simulink model "fwv_2020b"  (R2020b)
settings: Solver=ode15s  StartTime=0.0  StopTime=1  RelTol=1e-3  AbsTol=1e-3  EnableMultiTasking=on
model workspace: external: MATLAB File /home/jeff/文档/research/fwvlab/main.m (data not in the file)
values from neighbouring files (symbols this model uses):
  A_D = 1.5    [main.m]    (also in param.m; params.m)
  A_L = 1.8    [main.m]    (also in param.m; params.m)
  c_bar = S/R    (= 0.0357142857143)    [main.m]    (also in param.m = 0.0251327412287; params.m)
  C_D0 = 0.45    [main.m]    (also in param.m; params.m)
  m = 2    [rbf_pid.m]
  r00 = double(int(f,[0,1]))    [main.m]    (also in param.m = 1; params.m = 0.933333333333)
  r11 = double(int(x*f,[0,1]))    [main.m]    (also in param.m = double(int(curv(x)*(x+1/9),0,1)); params.m = 0.481185185185)
  r22 = double(int(x^2*f,[0,1]))    [main.m]    (also in param.m = double(int(curv(x)*(x+1/9)^2,0,1)); params.m = 0.304750617284)
  r33 = double(int(x^3*f,[0,1]))    [main.m]    (also in param.m = double(int(curv(x)*(x+1/9)^3,0,1)); params.m = 0.218568691358)
  r_cp = Rw*r33/r22    [main.m]    (also in param.m; params.m = 0.10758076225)
  rho = 1.205    [main.m]    (also in param.m; params.m)
  Rw = 0.15    [main.m]    (also in param.m = 0.075; params.m)
  z0 = double(int(f^2,[0,1]))    [main.m]
  z1 = double(int(x*f^2,[0,1]))    [main.m]
  z2 = double(int(x^2*f^2,[0,1]))    [main.m]
undefined symbols (not defined in the file or in its folder): X, Y, Z
libraries: sm_lib x45, nesl_utility x38
(part 1 of 2)
settings Model: OrderedModelArguments=off  Creator=jeff  LastModifiedBy=jeff
settings SolverCC: AutoScaleAbsTol=off
settings DataIOCC: LimitDataPoints=on  MaxDataPoints=10000
settings OptimizationCC: LifeSpan=inf
settings DebuggingCC: AllowSymbolicDim=off  SFUnexpectedBacktrackingDiag=warning  SFNoUnconditionalDefaultTransitionDiag=warning  SFExecutionAtInitializationDiag=none  ArithmeticOperatorsInVariantConditions=warning
settings ModelReferenceCC: ModelReferenceMinAlgLoopOccurrences=on
settings SFSimCC: SimUseLocalCustomCode=off  CustomCodeUndefinedFunction=UseInterfaceOnly
settings RTWCC: RTWUseLocalCustomCode=off
settings CodeAppCC: StateflowObjectComments=on
settings GRTTargetCC: TargetLangStandard=C89/C90 (ANSI)
settings ConfigComp: CovMetricSettings=dw  CovSaveCumulativeToWorkspaceVar=on  CovSaveSingleToWorkspaceVar=on  CovExternalEMLEnable=off  CovSFcnEnable=off
settings SimscapeCC: SimscapeLogType=all  SimscapeLogSimulationStatistics=on  SimscapeLogDataHistory=10000

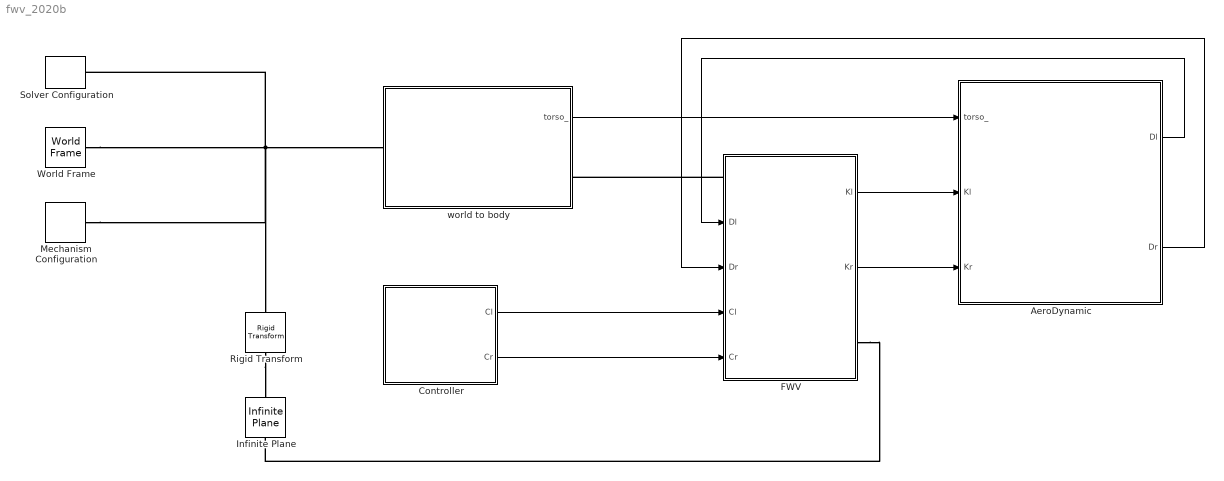
== system fwv_2020b ==
  AeroDynamic : Subsystem
  Controller : Subsystem  mask{f1=20}
  FWV : Subsystem  mask{rho_w=800, stif_rot=5e-3, stif_m=100, damp_m=10}
      settings: PortSchema="{\"entries\":[{\"content\":{\"sides\":[{\"content\":{\"connectorIds\":[\"LConn1\",\"In1\",\"In2\",\"In3\",\"In4\"]},\"type\":\"ConnectorPlacement.EquallySpacedRectSide\",\"uuid\":\"10a6bb1b-48cb-4367-84fe-ad8804c4af6f\"},{\"content\":{\"connectorIds\":[\"Out1\",\"Out2\",\"RConn1\"],\"side\":\"RIGHT\"},\"type\":\"ConnectorPlacement.EquallySpacedRectSide\",\"uuid\":\"a1c0f7ef-a6bf-4be1-8074-dff1a8dbc5c8\"},{\"content\":{\"connectorIds\":[],\"side\":\"TOP\"},\"type\":\"ConnectorPlacement.EquallySpacedRectSide\",\"uuid\":\"74d65e1b-e014-4639-84e4-d97080944fae\"}]},\"type\":\"ConnectorPlacement.EquallySpacedConnector\",\"uuid\":\"e5531aaa-1ccc-4e57-b614-20b26b45530b\"}],\"packageUris\":[\"http://schema.mathworks.com/mf0/Connector/R2020b\"],\"version\":\"1.0\"}"
  Infinite Plane : sm_lib/Curves and Surfaces/Infinite Plane  GraphicType=Rectangle  GraphicPlaneWidth=50  GraphicPlaneWidthUnits=m  GraphicPlaneHeight=50  GraphicPlaneHeightUnits=m  GraphicVisPropType=SimpleVisualProperties  GraphicDiffuseColor=[0.2 0.5 0.8]  GraphicOpacity=1  GraphicSpecularColor=[0.5 0.5 0.5 1.0]  GraphicAmbientColor=[0.15 0.15 0.15 1.0]  GraphicEmissiveColor=[0.0 0.0 0.0 1.0]  GraphicShininess=75
  Mechanism Configuration : sm_lib/Utilities/Mechanism Configuration  UniformGravity=Constant  GravityVector=[0 0 -9.80665]  GravityVectorUnits=m/s^2  GravityUnits=m/s^2  LinearizationDelta=0.001  JointModeTransitionNonlinearIterations=2
  Rigid Transform : sm_lib/Frames and Transforms/Rigid Transform  TranslationMethod=StandardAxis  TranslationStandardOffset=6.5  TranslationLengthUnit=cm  TranslationStandardAxis=-Z  TranslationCartesianOffset=[0 0 0]  TranslationROffset=0  TranslationROffsetUnits=m  TranslationZOffset=0  TranslationZOffsetUnits=m  TranslationThetaOffset=0  TranslationThetaOffsetUnits=deg  RotationMethod=None  RotationAngleUnits=deg  RotationStandardAxis=+Z  RotationAngle=0.0  RotationArbitraryAxis=[0 0 1]  FollAlignAxisA=+X  BaseAlignAxisA=+Y  FollAlignAxisB=+Y  BaseAlignAxisB=+Z  RotationSequenceAxes=FollowerAxes  RotationSequence=XYX  RotationSequenceAngles=[0 0 0]  RotationSequenceAnglesUnits=deg  RotationMatrix=[1 0 0; 0 1 0; 0 0 1]
  Solver Configuration : nesl_utility/Solver Configuration  PhysicalDomain=network_engine_domain  SubClassName=solver  LeftPortType=input  RightPortType=generic  Tones=[]  Harmonics=[]  SimulateNoise=off  Profile=off  UseLocalSampling=off  EnableSwitchedLinearOptims=on  FrequencyDomain=off  UseCCode=off  RelTol=0.001  AbsTol=1e-06  MinStep=1e-09  ToWorkspace=off  RevertToSquareIcSolve=off  NumHomotopyIterations=100  PhasorMode=off  PhasorModeNumHarmonics=1  DoDC=off  ResidualTolerance=1e-09  UseLocalSolver=off  LocalSolverChoice=NE_BACKWARD_EULER_ADVANCER  LocalSolverSampleTime=0.001  DoFixedCost=off  MaxNonlinIter=3  MaxModeIter=2  ComputeImpulses=off  ImpulseIterations=2  LinearAlgebra=Sparse  EquationFormulation=NE_TIME_EF  DelaysMemoryBudget=1024  AutomaticFiltering=on  FilteringTimeConstant=0.001  PartitionStorageMethod=AS_NEEDED  PartitionMemoryBudget=1024  PartitionMethod=FAST
      settings: SourceProductBaseCode=PW,SS
  World Frame : sm_lib/Frames and Transforms/World Frame
  world to body : Subsystem
  wires:
  world to body/1(torso_) -> AeroDynamic/1(torso_)
  FWV/1(Kl) -> AeroDynamic/2(Kl)
  FWV/2(Kr) -> AeroDynamic/3(Kr)
  Controller/1(Cl) -> FWV/3(Cl)
  Controller/2(Cr) -> FWV/4(Cr)
  AeroDynamic/2(Dr) -> FWV/2(Dr)
  AeroDynamic/1(Dl) -> FWV/1(Dl)
  connections:
  Rigid Transform/RConn1 -- Infinite Plane/LConn1
  FWV/RConn1 -- Infinite Plane/RConn1
  FWV/LConn1 -- world to body/RConn1
  World Frame/RConn1 -- world to body/LConn1 -- Mechanism Configuration/RConn1 -- Rigid Transform/LConn1 -- Solver Configuration/RConn1

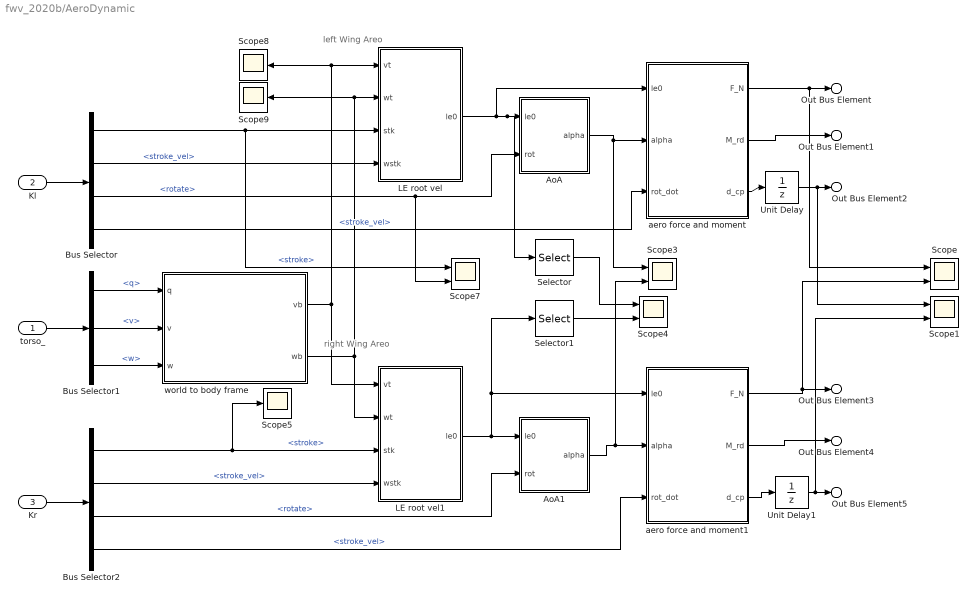
== system fwv_2020b/AeroDynamic ==
  note: right Wing Areo
  note: left Wing Areo
  torso_ : Inport
  Kl : Inport  Port=2
  Kr : Inport  Port=3
  AoA : MATLAB Function  TreatAsAtomicUnit=on
  AoA1 : MATLAB Function  TreatAsAtomicUnit=on
  Bus Selector : BusSelector  OutputSignals=stroke,stroke_vel,rotate,stroke_vel
  Bus Selector1 : BusSelector  OutputSignals=q,v,w
  Bus Selector2 : BusSelector  OutputSignals=stroke,stroke_vel,rotate,stroke_vel
  LE root vel : MATLAB Function  TreatAsAtomicUnit=on
  LE root vel1 : MATLAB Function  TreatAsAtomicUnit=on
  Scope{,1,3..4,7} (5 alike) : Scope  NumInputPorts=2
  Scope5 : Scope
  Scope8 : Scope
  Scope9 : Scope
  Selector : Selector  NumberOfDimensions=2  InputPortWidth=3  IndexOptions=Starting index (dialog),Starting index (dialog)  Indices=2,1  OutputSizes=1,1
  Selector1 : Selector  NumberOfDimensions=2  InputPortWidth=3  IndexOptions=Index vector (dialog),Index vector (dialog)  Indices=2,1  OutputSizes=1,1
  Unit Delay : UnitDelay  InitialCondition=-0.51*c_bar  SampleTime=-1  HasFrameUpgradeWarning=on
  Unit Delay1 : UnitDelay  InitialCondition=-0.51*c_bar  SampleTime=-1  HasFrameUpgradeWarning=on
  aero force and moment : MATLAB Function  TreatAsAtomicUnit=on
  aero force and moment1 : MATLAB Function  TreatAsAtomicUnit=on
  world to body frame : MATLAB Function  TreatAsAtomicUnit=on
  Out Bus Element : Outport  PortName=Dl  Element=FN
  Out Bus Element1 : Outport  PortName=Dl  Element=My
  Out Bus Element2 : Outport  PortName=Dl  Element=d_cp
  Out Bus Element3 : Outport  Port=2  PortName=Dr  Element=FN
  Out Bus Element4 : Outport  Port=2  PortName=Dr  Element=My
  Out Bus Element5 : Outport  Port=2  PortName=Dr  Element=d_cp
  wires:
  AoA/1(alpha) -> Scope3/1, aero force and moment/2(alpha)
  Kl/1 -> Bus Selector/1
  Bus Selector/1 -> Scope7/1, LE root vel/3(stk)  "<stroke>"
  Bus Selector/2 -> LE root vel/4(wstk)  "<stroke_vel>"
  torso_/1 -> Bus Selector1/1
  Bus Selector/3 -> Scope7/2, AoA/2(rot)  "<rotate>"
  Bus Selector1/1 -> world to body frame/1(q)  "<q>"
  Bus Selector1/2 -> world to body frame/2(v)  "<v>"
  Bus Selector1/3 -> world to body frame/3(w)  "<w>"
  world to body frame/1(vb) -> Scope8/1, LE root vel/1(vt), LE root vel1/1(vt)
  world to body frame/2(wb) -> Scope9/1, LE root vel/2(wt), LE root vel1/2(wt)
  LE root vel/1(le0) -> Selector/1, AoA/1(le0), aero force and moment/1(le0)
  aero force and moment/2(M_rd) -> Out Bus Element1/1
  aero force and moment/3(d_cp) -> Unit Delay/1
  Kr/1 -> Bus Selector2/1
  aero force and moment1/2(M_rd) -> Out Bus Element4/1
  aero force and moment1/3(d_cp) -> Unit Delay1/1
  LE root vel1/1(le0) -> Selector1/1, aero force and moment1/1(le0), AoA1/1(le0)
  Bus Selector2/3 -> AoA1/2(rot)  "<rotate>"
  Bus Selector2/1 -> Scope5/1, LE root vel1/3(stk)  "<stroke>"
  Bus Selector2/2 -> LE root vel1/4(wstk)  "<stroke_vel>"
  AoA1/1(alpha) -> Scope3/2, aero force and moment1/2(alpha)
  Bus Selector/4 -> aero force and moment/3(rot_dot)  "<stroke_vel>"
  Bus Selector2/4 -> aero force and moment1/3(rot_dot)  "<stroke_vel>"
  aero force and moment/1(F_N) -> Out Bus Element/1, Scope/1
  aero force and moment1/1(F_N) -> Scope/2, Out Bus Element3/1
  Selector/1 -> Scope4/1
  Selector1/1 -> Scope4/2
  Unit Delay1/1 -> Scope1/2, Out Bus Element5/1
  Unit Delay/1 -> Scope1/1, Out Bus Element2/1

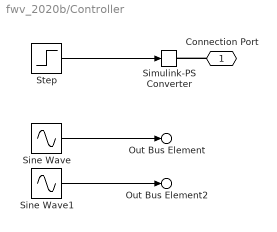
== system fwv_2020b/Controller ==
  Simulink-PS Converter : nesl_utility/Simulink-PS Converter  PhysicalDomain=network_engine_domain  SubClassName=ps_input  LeftPortType=input  RightPortType=output  PseudoPeriodic=off  Frequencies=[]  NoiseDistribution=none  NoiseParameters=[]  Unit=1  AffineConversion=off  FilteringAndDerivatives=provide  SimscapeFilterOrder=1  InputFilterTimeConstant=0.001  UdotUserProvided=0
      settings: SourceProductBaseCode=PW,SS
  Sine Wave : Sin  Amplitude=pi/3  Frequency=f1*2*pi  SampleTime=0
  Sine Wave1 : Sin  Amplitude=pi/3  Frequency=f1*2*pi  SampleTime=0
  Step : Step  Time=0.09  After=-1  SampleTime=0
  Connection Port : PMIOPort  Side=Left
  Out Bus Element : Outport  PortName=Cl  Element=stroke
  Out Bus Element2 : Outport  Port=2  PortName=Cr  Element=stroke
  wires:
  Sine Wave/1 -> Out Bus Element/1
  Sine Wave1/1 -> Out Bus Element2/1
  Step/1 -> Simulink-PS Converter/1
  connections:
  Connection Port/RConn1 -- Simulink-PS Converter/RConn1

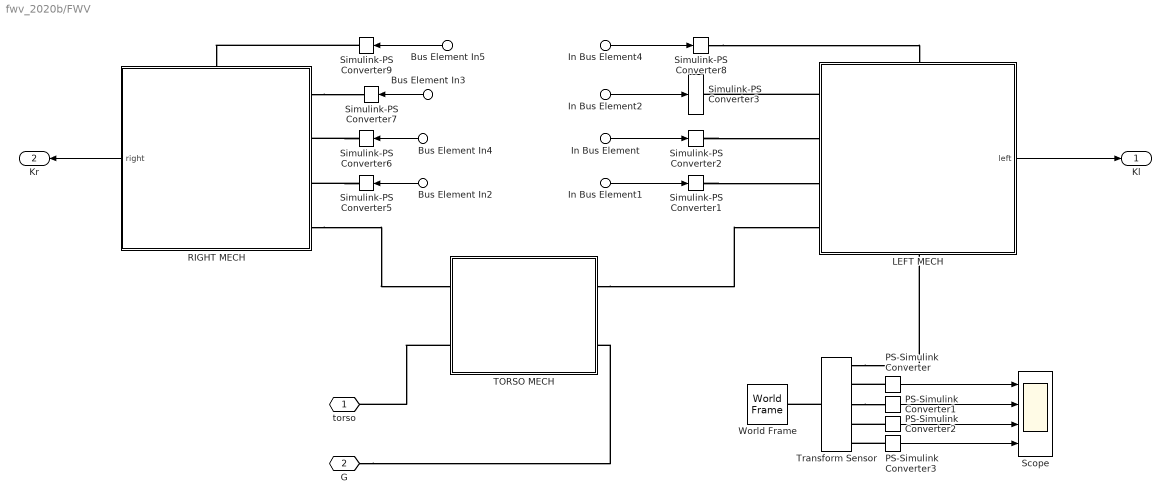
== system fwv_2020b/FWV ==
  In Bus Element : Inport  PortName=Dl  Element=FN
  In Bus Element1 : Inport  PortName=Dl  Element=My
  In Bus Element4 : Inport  PortName=Dl  Element=d_cp
  Bus Element In4 : Inport  Port=2  PortName=Dr  Element=FN
  Bus Element In2 : Inport  Port=2  PortName=Dr  Element=My
  Bus Element In5 : Inport  Port=2  PortName=Dr  Element=d_cp
  In Bus Element2 : Inport  Port=3  PortName=Cl  Element=stroke
  Bus Element In3 : Inport  Port=4  PortName=Cr  Element=stroke
  LEFT MECH : Subsystem
      settings: PortSchema="{\"entries\":[{\"content\":{\"sides\":[{\"content\":{\"connectorIds\":[\"LConn1\",\"LConn2\",\"LConn3\",\"LConn4\"]},\"type\":\"ConnectorPlacement.EquallySpacedRectSide\",\"uuid\":\"3b3bd30c-9c3d-4020-920e-73dfb95645be\"},{\"content\":{\"connectorIds\":[\"Out1\"],\"side\":\"RIGHT\"},\"type\":\"ConnectorPlacement.EquallySpacedRectSide\",\"uuid\":\"6bf80106-81c9-4f1a-b6c7-4ab6b75d5951\"},{\"content\":{\"connectorIds\":[\"LConn5\"],\"side\":\"TOP\"},\"type\":\"ConnectorPlacement.EquallySpacedRectSide\",\"uuid\":\"ce1b4233-3217-452e-b464-d84889ce50ed\"},{\"content\":{\"connectorIds\":[\"RConn1\"],\"side\":\"BOTTOM\"},\"type\":\"ConnectorPlacement.EquallySpacedRectSide\",\"uuid\":\"0b387201-862b-4d94-b297-724f4b58a817\"}]},\"type\":\"ConnectorPlacement.EquallySpacedConnector\",\"uuid\":\"4ad9753c-a95f-426b-a419-920792cb5c12\"}],\"packageUris\":[\"http://schema.mathworks.com/mf0/Connector/R2020b\"],\"version\":\"1.0\"}"
  PS-Simulink Converter{,1..3} (4 alike) : nesl_utility/PS-Simulink Converter  PhysicalDomain=network_engine_domain  SubClassName=ps_output  LeftPortType=input  RightPortType=output  PseudoPeriodic=off  Frequencies=[]  Unit=inherit  AffineConversion=off
      settings: SourceProductBaseCode=PW,SS
  RIGHT MECH : Subsystem
      settings: PortSchema="{\"entries\":[{\"content\":{\"sides\":[{\"content\":{\"connectorIds\":[\"LConn1\",\"LConn2\",\"LConn3\",\"LConn4\"]},\"type\":\"ConnectorPlacement.EquallySpacedRectSide\",\"uuid\":\"3b3bd30c-9c3d-4020-920e-73dfb95645be\"},{\"content\":{\"connectorIds\":[\"Out1\"],\"side\":\"RIGHT\"},\"type\":\"ConnectorPlacement.EquallySpacedRectSide\",\"uuid\":\"6bf80106-81c9-4f1a-b6c7-4ab6b75d5951\"},{\"content\":{\"connectorIds\":[\"LConn5\"],\"side\":\"TOP\"},\"type\":\"ConnectorPlacement.EquallySpacedRectSide\",\"uuid\":\"ce1b4233-3217-452e-b464-d84889ce50ed\"},{\"content\":{\"connectorIds\":[],\"side\":\"BOTTOM\"},\"type\":\"ConnectorPlacement.EquallySpacedRectSide\",\"uuid\":\"e55bd33d-a165-4775-a049-8f5077b03cfa\"}]},\"type\":\"ConnectorPlacement.EquallySpacedConnector\",\"uuid\":\"4ad9753c-a95f-426b-a419-920792cb5c12\"}],\"packageUris\":[\"http://schema.mathworks.com/mf0/Connector/R2020b\"],\"version\":\"1.0\"}"
  Scope : Scope  NumInputPorts=4
  Simulink-PS Converter{1..2,5..9} (7 alike) : nesl_utility/Simulink-PS Converter  PhysicalDomain=network_engine_domain  SubClassName=ps_input  LeftPortType=input  RightPortType=output  PseudoPeriodic=off  Frequencies=[]  NoiseDistribution=none  NoiseParameters=[]  Unit=1  AffineConversion=off  FilteringAndDerivatives=filter  SimscapeFilterOrder=2  InputFilterTimeConstant=0.001  UdotUserProvided=0
      settings: SourceProductBaseCode=PW,SS
  Simulink-PS Converter3 : nesl_utility/Simulink-PS Converter  PhysicalDomain=network_engine_domain  SubClassName=ps_input  LeftPortType=input  RightPortType=output  PseudoPeriodic=off  Frequencies=[]  NoiseDistribution=none  NoiseParameters=[]  Unit=1  AffineConversion=off  FilteringAndDerivatives=filter  SimscapeFilterOrder=2  InputFilterTimeConstant=0.001  UdotUserProvided=2
      settings: SourceProductBaseCode=PW,SS
  TORSO MECH : Subsystem  mask{mu0=0, mu1=0}
  Transform Sensor : sm_lib/Frames and Transforms/Transform Sensor  MeasurementFrame=NonRotatingFollower  SenseAngle=off  SenseAxis=off  SenseAngle1=off  SenseAngle2=off  SenseAngle3=off  SenseQ=off  SenseR=off  SenseOmegaX=on  SenseOmegaY=off  SenseOmegaZ=on  SenseOmega1=off  SenseOmega2=off  SenseOmega3=off  SenseQDot=off  SenseRDot=off  SenseAlphaX=off  SenseAlphaY=off  SenseAlphaZ=off  SenseAlpha1=off  SenseAlpha2=off  SenseAlpha3=off  SenseQDDot=off  SenseRDDot=off  SenseX=off  SenseY=off  SenseZ=off  SenseRad=off  SenseAzim=off  SenseDist=off  SenseInc=off  SenseXDot=on  SenseYDot=off  SenseZDot=on  SenseRadDot=off  SenseAzimDot=off  SenseDistDot=off  SenseIncDot=off  SenseXDDot=off  SenseYDDot=off  SenseZDDot=off  SenseRadDDot=off  SenseAzimDDot=off  SenseDistDDot=off  SenseIncDDot=off
  World Frame : sm_lib/Frames and Transforms/World Frame
  torso : PMIOPort  Side=Left
  G : PMIOPort  Port=2  Side=Right
  Kl : Outport
  Kr : Outport  Port=2
  wires:
  LEFT MECH/1(left) -> Kl/1
  RIGHT MECH/1(right) -> Kr/1
  In Bus Element1/1 -> Simulink-PS Converter1/1
  In Bus Element/1 -> Simulink-PS Converter2/1
  In Bus Element2/1 -> Simulink-PS Converter3/1
  Bus Element In3/1 -> Simulink-PS Converter7/1
  Bus Element In4/1 -> Simulink-PS Converter6/1
  Bus Element In2/1 -> Simulink-PS Converter5/1
  In Bus Element4/1 -> Simulink-PS Converter8/1
  Bus Element In5/1 -> Simulink-PS Converter9/1
  PS-Simulink Converter/1 -> Scope/1
  PS-Simulink Converter1/1 -> Scope/2
  PS-Simulink Converter2/1 -> Scope/3
  PS-Simulink Converter3/1 -> Scope/4
  connections:
  G/RConn1 -- TORSO MECH/RConn2
  TORSO MECH/LConn2 -- torso/RConn1
  TORSO MECH/RConn1 -- LEFT MECH/LConn4
  RIGHT MECH/LConn4 -- TORSO MECH/LConn1
  LEFT MECH/LConn1 -- Simulink-PS Converter3/RConn1
  RIGHT MECH/LConn1 -- Simulink-PS Converter7/RConn1
  Simulink-PS Converter2/RConn1 -- LEFT MECH/LConn2
  Simulink-PS Converter1/RConn1 -- LEFT MECH/LConn3
  Simulink-PS Converter6/RConn1 -- RIGHT MECH/LConn2
  Simulink-PS Converter5/RConn1 -- RIGHT MECH/LConn3
  Simulink-PS Converter8/RConn1 -- LEFT MECH/LConn5
  Simulink-PS Converter9/RConn1 -- RIGHT MECH/LConn5
  Transform Sensor/LConn1 -- World Frame/RConn1
  Transform Sensor/RConn1 -- LEFT MECH/RConn1
  PS-Simulink Converter/LConn1 -- Transform Sensor/RConn2
  Transform Sensor/RConn3 -- PS-Simulink Converter1/LConn1
  PS-Simulink Converter2/LConn1 -- Transform Sensor/RConn4
  PS-Simulink Converter3/LConn1 -- Transform Sensor/RConn5

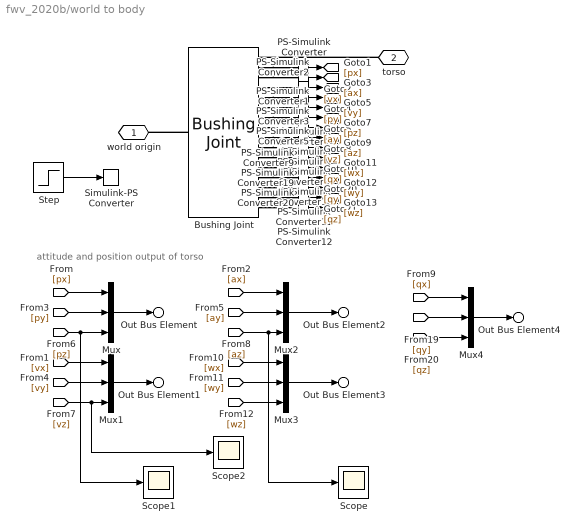
== system fwv_2020b/world to body ==
  note: attitude and position output of torso
  Bushing Joint : sm_lib/Joints/Bushing Joint  JointMode=Normal  SenseConstraintForce=off  SenseConstraintForceX=off  SenseConstraintForceY=off  SenseConstraintForceZ=off  SenseConstraintTorque=off  SenseConstraintTorqueX=off  SenseConstraintTorqueY=off  SenseConstraintTorqueZ=off  SenseTotalForce=off  SenseTotalForceX=off  SenseTotalForceY=off  SenseTotalForceZ=off  SenseTotalTorque=off  SenseTotalTorqueX=off  SenseTotalTorqueY=off  SenseTotalTorqueZ=off  CompositeWrenchDir=FollowerOnBase  CompositeWrenchFrame=BaseFrame  PxEquilibriumPosition=0  PxEquilibriumPositionUnits=m  PxSpringStiffness=0  PxSpringStiffnessUnits=N/m  PxDampingCoefficient=0  PxDampingCoefficientUnits=N/(m/s)  PxTorqueActuationMode=NoTorque  PxMotionActuationMode=ComputedMotion  PxSensePosition=on  PxSenseVelocity=on  PxSenseAcceleration=on  PxSenseTorqueForce=off  PxSenseLowerLimitTorqueForce=off  PxSenseUpperLimitTorqueForce=off  PxLowerLimitSpecify=off  PxLowerLimitBound=-1  PxLowerLimitBoundUnits=m  PxLowerLimitStiffness=1e6  PxLowerLimitStiffnessUnits=N/m  PxLowerLimitDamping=1e3  PxLowerLimitDampingUnits=N/(m/s)  PxLowerLimitTransitionRegionWidth=1e-4  PxLowerLimitTransitionRegionWidthUnits=m  PxUpperLimitSpecify=off  PxUpperLimitBound=1  PxUpperLimitBoundUnits=m  PxUpperLimitStiffness=1e6  PxUpperLimitStiffnessUnits=N/m  PxUpperLimitDamping=1e3  PxUpperLimitDampingUnits=N/(m/s)  PxUpperLimitTransitionRegionWidth=1e-4  PxUpperLimitTransitionRegionWidthUnits=m  PxPositionTargetSpecify=off  PxPositionTargetPriority=High  PxPositionTargetValue=0  PxPositionTargetValueUnits=m  PxVelocityTargetSpecify=off  PxVelocityTargetPriority=High  PxVelocityTargetValue=0  PxVelocityTargetValueUnits=m/s  PyEquilibriumPosition=0  PyEquilibriumPositionUnits=m  PySpringStiffness=0  PySpringStiffnessUnits=N/m  PyDampingCoefficient=0  PyDampingCoefficientUnits=N/(m/s)  PyTorqueActuationMode=NoTorque  PyMotionActuationMode=ComputedMotion  PySensePosition=on  PySenseVelocity=on  PySenseAcceleration=on  PySenseTorqueForce=off  PySenseLowerLimitTorqueForce=off  PySenseUpperLimitTorqueForce=off  PyLowerLimitSpecify=off  PyLowerLimitBound=-1  PyLowerLimitBoundUnits=m  PyLowerLimitStiffness=1e6  PyLowerLimitStiffnessUnits=N/m  PyLowerLimitDamping=1e3  PyLowerLimitDampingUnits=N/(m/s)  PyLowerLimitTransitionRegionWidth=1e-4  PyLowerLimitTransitionRegionWidthUnits=m  PyUpperLimitSpecify=off  PyUpperLimitBound=1  PyUpperLimitBoundUnits=m  PyUpperLimitStiffness=1e6  PyUpperLimitStiffnessUnits=N/m  PyUpperLimitDamping=1e3  PyUpperLimitDampingUnits=N/(m/s)  PyUpperLimitTransitionRegionWidth=1e-4  PyUpperLimitTransitionRegionWidthUnits=m  PyPositionTargetSpecify=off  PyPositionTargetPriority=High  PyPositionTargetValue=0  PyPositionTargetValueUnits=m  PyVelocityTargetSpecify=off  PyVelocityTargetPriority=High  PyVelocityTargetValue=0  PyVelocityTargetValueUnits=m/s  PzEquilibriumPosition=0  PzEquilibriumPositionUnits=m  PzSpringStiffness=0  PzSpringStiffnessUnits=N/m  PzDampingCoefficient=0  PzDampingCoefficientUnits=N/(m/s)  PzTorqueActuationMode=NoTorque  PzMotionActuationMode=ComputedMotion  PzSensePosition=on  PzSenseVelocity=on  PzSenseAcceleration=on  PzSenseTorqueForce=off  PzSenseLowerLimitTorqueForce=off  PzSenseUpperLimitTorqueForce=off  PzLowerLimitSpecify=off  PzLowerLimitBound=-1  PzLowerLimitBoundUnits=m  PzLowerLimitStiffness=1e6  PzLowerLimitStiffnessUnits=N/m  PzLowerLimitDamping=1e3  PzLowerLimitDampingUnits=N/(m/s)  PzLowerLimitTransitionRegionWidth=1e-4  PzLowerLimitTransitionRegionWidthUnits=m  PzUpperLimitSpecify=off  PzUpperLimitBound=1  PzUpperLimitBoundUnits=m  PzUpperLimitStiffness=1e6  PzUpperLimitStiffnessUnits=N/m  PzUpperLimitDamping=1e3  PzUpperLimitDampingUnits=N/(m/s)  PzUpperLimitTransitionRegionWidth=1e-4  PzUpperLimitTransitionRegionWidthUnits=m  PzPositionTargetSpecify=off  PzPositionTargetPriority=High  PzPositionTargetValue=0  PzPositionTargetValueUnits=m  PzVelocityTargetSpecify=off  PzVelocityTargetPriority=High  PzVelocityTargetValue=0  PzVelocityTargetValueUnits=m/s  RxEquilibriumPosition=0  RxEquilibriumPositionUnits=deg  RxSpringStiffness=0  RxSpringStiffnessUnits=N*m/deg  RxDampingCoefficient=0  RxDampingCoefficientUnits=N*m/(deg/s)  RxTorqueActuationMode=NoTorque  RxMotionActuationMode=ComputedMotion  RxSensePosition=on  RxSenseVelocity=on  RxSenseAcceleration=off  RxSenseTorqueForce=off  RxSenseLowerLimitTorqueForce=off  RxSenseUpperLimitTorqueForce=off  RxLowerLimitSpecify=off  RxLowerLimitBound=-90  RxLowerLimitBoundUnits=deg  RxLowerLimitStiffness=1e4  RxLowerLimitStiffnessUnits=N*m/deg  RxLowerLimitDamping=10  RxLowerLimitDampingUnits=N*m/(deg/s)  RxLowerLimitTransitionRegionWidth=0.1  RxLowerLimitTransitionRegionWidthUnits=deg  RxUpperLimitSpecify=off  RxUpperLimitBound=90  RxUpperLimitBoundUnits=deg  RxUpperLimitStiffness=1e4  RxUpperLimitStiffnessUnits=N*m/deg  RxUpperLimitDamping=10  RxUpperLimitDampingUnits=N*m/(deg/s)  RxUpperLimitTransitionRegionWidth=0.1  RxUpperLimitTransitionRegionWidthUnits=deg  RxPositionTargetSpecify=off  RxPositionTargetPriority=High  RxPositionTargetValue=0  RxPositionTargetValueUnits=deg  RxVelocityTargetSpecify=off  RxVelocityTargetPriority=High  RxVelocityTargetValue=0  RxVelocityTargetValueUnits=deg/s  RyEquilibriumPosition=0  RyEquilibriumPositionUnits=deg  RySpringStiffness=0  RySpringStiffnessUnits=N*m/deg  RyDampingCoefficient=0  RyDampingCoefficientUnits=N*m/(deg/s)  RyTorqueActuationMode=NoTorque  RyMotionActuationMode=ComputedMotion  RySensePosition=on  RySenseVelocity=on  RySenseAcceleration=off  RySenseTorqueForce=off  RySenseLowerLimitTorqueForce=off  RySenseUpperLimitTorqueForce=off  RyLowerLimitSpecify=off  RyLowerLimitBound=-90  RyLowerLimitBoundUnits=deg  RyLowerLimitStiffness=1e4  RyLowerLimitStiffnessUnits=N*m/deg  RyLowerLimitDamping=10  RyLowerLimitDampingUnits=N*m/(deg/s)  RyLowerLimitTransitionRegionWidth=0.1  RyLowerLimitTransitionRegionWidthUnits=deg  RyUpperLimitSpecify=off  RyUpperLimitBound=90  RyUpperLimitBoundUnits=deg  RyUpperLimitStiffness=1e4  RyUpperLimitStiffnessUnits=N*m/deg  RyUpperLimitDamping=10  RyUpperLimitDampingUnits=N*m/(deg/s)  RyUpperLimitTransitionRegionWidth=0.1  RyUpperLimitTransitionRegionWidthUnits=deg  RyPositionTargetSpecify=off  RyPositionTargetPriority=High  RyPositionTargetValue=0  RyPositionTargetValueUnits=deg  RyVelocityTargetSpecify=off  RyVelocityTargetPriority=High  RyVelocityTargetValue=0  RyVelocityTargetValueUnits=deg/s  RzEquilibriumPosition=0  RzEquilibriumPositionUnits=deg  RzSpringStiffness=0  RzSpringStiffnessUnits=N*m/deg  RzDampingCoefficient=0  RzDampingCoefficientUnits=N*m/(deg/s)  RzTorqueActuationMode=NoTorque  RzMotionActuationMode=ComputedMotion  RzSensePosition=on  RzSenseVelocity=on  RzSenseAcceleration=off  RzSenseTorqueForce=off  RzSenseLowerLimitTorqueForce=off  RzSenseUpperLimitTorqueForce=off  RzLowerLimitSpecify=off  RzLowerLimitBound=-90  RzLowerLimitBoundUnits=deg  RzLowerLimitStiffness=1e4  RzLowerLimitStiffnessUnits=N*m/deg  RzLowerLimitDamping=10  RzLowerLimitDampingUnits=N*m/(deg/s)  RzLowerLimitTransitionRegionWidth=0.1  RzLowerLimitTransitionRegionWidthUnits=deg  RzUpperLimitSpecify=off  RzUpperLimitBound=90  RzUpperLimitBoundUnits=deg  RzUpperLimitStiffness=1e4  RzUpperLimitStiffnessUnits=N*m/deg  RzUpperLimitDamping=10  RzUpperLimitDampingUnits=N*m/(deg/s)  RzUpperLimitTransitionRegionWidth=0.1  RzUpperLimitTransitionRegionWidthUnits=deg  RzPositionTargetSpecify=off  RzPositionTargetPriority=High  RzPositionTargetValue=45  RzPositionTargetValueUnits=deg  RzVelocityTargetSpecify=off  RzVelocityTargetPriority=High  RzVelocityTargetValue=0  RzVelocityTargetValueUnits=deg/s
  Mux{,1..4} (5 alike) : Mux  Inputs=3
  PS-Simulink Converter{,1..12,19..20} (15 alike) : nesl_utility/PS-Simulink Converter  PhysicalDomain=network_engine_domain  SubClassName=ps_output  LeftPortType=input  RightPortType=output  PseudoPeriodic=off  Frequencies=[]  Unit=inherit  AffineConversion=off
      settings: SourceProductBaseCode=PW,SS
  Scope : Scope
  Scope1 : Scope
  Scope2 : Scope
  Simulink-PS Converter : nesl_utility/Simulink-PS Converter  PhysicalDomain=network_engine_domain  SubClassName=ps_input  LeftPortType=input  RightPortType=output  PseudoPeriodic=off  Frequencies=[]  NoiseDistribution=none  NoiseParameters=[]  Unit=1  AffineConversion=off  FilteringAndDerivatives=provide  SimscapeFilterOrder=1  InputFilterTimeConstant=0.001  UdotUserProvided=0
      settings: SourceProductBaseCode=PW,SS
  Step : Step  Time=0.5  After=0  SampleTime=0
  world origin : PMIOPort  Side=Left
  torso : PMIOPort  Port=2  Side=Right
  Out Bus Element : Outport  PortName=torso_  Element=p
  Out Bus Element1 : Outport  PortName=torso_  Element=v
  Out Bus Element2 : Outport  PortName=torso_  Element=a
  Out Bus Element3 : Outport  PortName=torso_  Element=w
  Out Bus Element4 : Outport  PortName=torso_  Element=q
  wires:
  PS-Simulink Converter10/1 -> [wx]
  PS-Simulink Converter9/1 -> [qx]
  [wz] -> Mux3/3
  [vy] -> Mux1/2
  [px] -> Mux/1
  [ax] -> Mux2/1
  [wx] -> Mux3/1
  PS-Simulink Converter8/1 -> [az]
  [vz] -> Scope2/1, Mux1/3
  Mux1/1 -> Out Bus Element1/1
  [az] -> Scope/1, Mux2/3
  PS-Simulink Converter5/1 -> [ay]
  [vx] -> Mux1/1
  [ay] -> Mux2/2
  PS-Simulink Converter7/1 -> [vz]
  [qy] -> Mux4/2
  [pz] -> Scope1/1, Mux/3
  Mux3/1 -> Out Bus Element3/1
  PS-Simulink Converter6/1 -> [pz]
  PS-Simulink Converter2/1 -> [ax]
  Mux/1 -> Out Bus Element/1
  Mux2/1 -> Out Bus Element2/1
  PS-Simulink Converter4/1 -> [vy]
  Mux4/1 -> Out Bus Element4/1
  PS-Simulink Converter/1 -> [px]
  PS-Simulink Converter3/1 -> [py]
  [py] -> Mux/2
  PS-Simulink Converter1/1 -> [vx]
  [wy] -> Mux3/2
  PS-Simulink Converter11/1 -> [wy]
  [qx] -> Mux4/1
  PS-Simulink Converter12/1 -> [wz]
  PS-Simulink Converter19/1 -> [qy]
  PS-Simulink Converter20/1 -> [qz]
  [qz] -> Mux4/3
  Step/1 -> Simulink-PS Converter/1
  connections:
  Bushing Joint/RConn3 -- PS-Simulink Converter1/LConn1
  Bushing Joint/RConn4 -- PS-Simulink Converter2/LConn1
  Bushing Joint/LConn1 -- world origin/RConn1
  Bushing Joint/RConn5 -- PS-Simulink Converter3/LConn1
  Bushing Joint/RConn9 -- PS-Simulink Converter7/LConn1
  Bushing Joint/RConn2 -- PS-Simulink Converter/LConn1
  Bushing Joint/RConn11 -- PS-Simulink Converter9/LConn1
  Bushing Joint/RConn15 -- PS-Simulink Converter20/LConn1
  Bushing Joint/RConn8 -- PS-Simulink Converter6/LConn1
  Bushing Joint/RConn10 -- PS-Simulink Converter8/LConn1
  Bushing Joint/RConn12 -- PS-Simulink Converter10/LConn1
  Bushing Joint/RConn16 -- PS-Simulink Converter12/LConn1
  Bushing Joint/RConn7 -- PS-Simulink Converter5/LConn1
  Bushing Joint/RConn14 -- PS-Simulink Converter11/LConn1
  Bushing Joint/RConn6 -- PS-Simulink Converter4/LConn1
  Bushing Joint/RConn13 -- PS-Simulink Converter19/LConn1
  torso/RConn1 -- Bushing Joint/RConn1

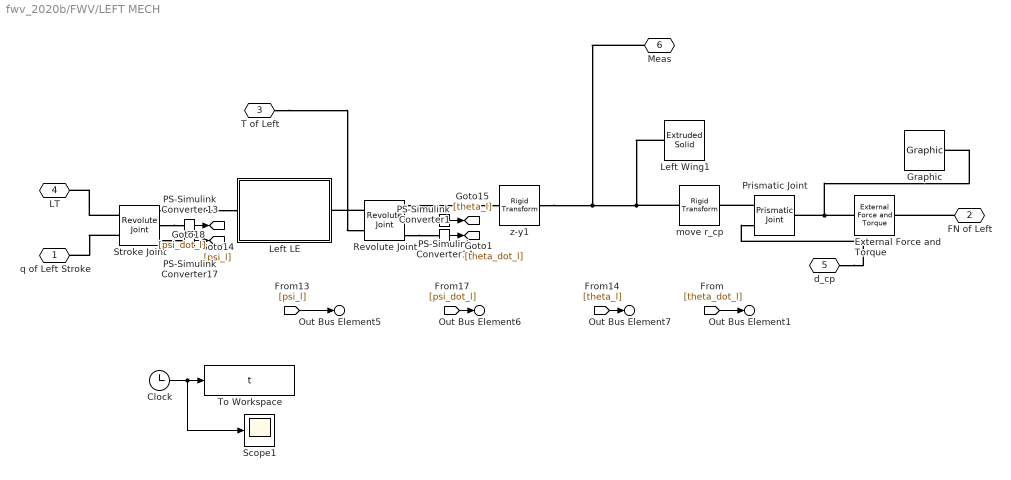
== system fwv_2020b/FWV/LEFT MECH ==
  Clock : Clock
  External Force and Torque : sm_lib/Forces and Torques/External Force and Torque  ForceResolutionFrame=AttachedFrame  EnableForceX=on  EnableForceY=off  EnableForceZ=off  EnableForce=off  TorqueResolutionFrame=AttachedFrame  EnableTorqueX=off  EnableTorqueY=off  EnableTorqueZ=off  EnableTorque=off
  Graphic : sm_lib/Body Elements/Graphic  GraphicType=Marker  MarkerShape=Frame  MarkerSize=20  GraphicVisPropType=SimpleVisualProperties  GraphicDiffuseColor=[1 0 1]  GraphicSpecularColor=[0.5 0.5 0.5 1.0]  GraphicAmbientColor=[0.15 0.15 0.15 1.0]  GraphicEmissiveColor=[0.0 0.0 0.0 1.0]  GraphicShininess=75  GraphicOpacity=1.0
  Left LE : Subsystem
  Left Wing1 : sm_lib/Body Elements/Extruded Solid  GraphicAmbientColor=[0.15 0.15 0.15 1.0]  BasedOnType=Density  CenterOfMass=[0 0 0]  CenterOfMassUnits=m  GraphicDiffuseColor=[0.5 0.5 0.5]  ExportConvexHullGeometry=off  ExtrusionCrossSection=[0 0; 20 -50; 140 -25; 140 0]  ExtrusionCrossSectionUnits=mm  Density=rho_w  DensityUnits=kg/m^3  DoExposeReferenceFrame=off  GraphicEmissiveColor=[0.0 0.0 0.0 1.0]  ExportEntireGeometry=off  ExtrusionLength=0.06  ExtrusionLengthUnits=mm  ExtrusionType=General  SerializedFrames=<Frames><Frame><Id>Frame1</Id><Value><Name>F1</Name><Origin><Source>ReferenceFrame</Source><FeatureName></FeatureName></Origin><PrimaryAxis><DefinedDirection>+X</DefinedDirection><Source>ReferenceFrame</Source><SourceDirection>+Z</SourceDirection><FeatureName></FeatureName></PrimaryAxis><SecondaryAxis><DefinedDirection>+Y</DefinedDirection><Source>ReferenceFrame</Source><SourceDirection>+X</SourceDirection><FeatureName></FeatureName></SecondaryAxis></Value></Frame></Frames>  MarkerShape=Sphere  MarkerSize=10  GraphicType=FromGeometry  InertiaType=CalculateFromGeometry  Mass=1  MassUnits=kg  MomentsOfInertia=[1 1 1]  MomentsOfInertiaUnits=kg*m^2  PolygonNumSides=3  GraphicOpacity=1.0  PolygonOuterRadius=1  PolygonOuterRadiusUnits=m  ProductsOfInertia=[0 0 0]  ProductsOfInertiaUnits=kg*m^2  GraphicShininess=75  GraphicSpecularColor=[0.5 0.5 0.5 1.0]  GraphicVisPropType=SimpleVisualProperties
  PS-Simulink Converter{1,13..14,17} (4 alike) : nesl_utility/PS-Simulink Converter  PhysicalDomain=network_engine_domain  SubClassName=ps_output  LeftPortType=input  RightPortType=output  PseudoPeriodic=off  Frequencies=[]  Unit=inherit  AffineConversion=off
      settings: SourceProductBaseCode=PW,SS
  Prismatic Joint : sm_lib/Joints/Prismatic Joint  JointMode=Normal  SenseConstraintForce=off  SenseConstraintForceX=off  SenseConstraintForceY=off  SenseConstraintForceZ=off  SenseConstraintTorque=off  SenseConstraintTorqueX=off  SenseConstraintTorqueY=off  SenseConstraintTorqueZ=off  SenseTotalForce=off  SenseTotalForceX=off  SenseTotalForceY=off  SenseTotalForceZ=off  SenseTotalTorque=off  SenseTotalTorqueX=off  SenseTotalTorqueY=off  SenseTotalTorqueZ=off  CompositeWrenchDir=FollowerOnBase  CompositeWrenchFrame=BaseFrame  EquilibriumPosition=0  EquilibriumPositionUnits=m  SpringStiffness=0  SpringStiffnessUnits=N/m  DampingCoefficient=0  DampingCoefficientUnits=N/(m/s)  TorqueActuationMode=ComputedTorque  MotionActuationMode=InputMotion  SensePosition=off  SenseVelocity=off  SenseAcceleration=off  SenseTorqueForce=off  SenseLowerLimitTorqueForce=off  SenseUpperLimitTorqueForce=off  LowerLimitSpecify=off  LowerLimitBound=-1  LowerLimitBoundUnits=m  LowerLimitStiffness=1e6  LowerLimitStiffnessUnits=N/m  LowerLimitDamping=1e3  LowerLimitDampingUnits=N/(m/s)  LowerLimitTransitionRegionWidth=1e-4  LowerLimitTransitionRegionWidthUnits=m  UpperLimitSpecify=off  UpperLimitBound=1  UpperLimitBoundUnits=m  UpperLimitStiffness=1e6  UpperLimitStiffnessUnits=N/m  UpperLimitDamping=1e3  UpperLimitDampingUnits=N/(m/s)  UpperLimitTransitionRegionWidth=1e-4  UpperLimitTransitionRegionWidthUnits=m  PositionTargetSpecify=off  PositionTargetPriority=High  PositionTargetValue=0  PositionTargetValueUnits=m  VelocityTargetSpecify=off  VelocityTargetPriority=High  VelocityTargetValue=0  VelocityTargetValueUnits=m/s
  Revolute Joint : sm_lib/Joints/Revolute Joint  JointMode=Normal  SenseConstraintForce=off  SenseConstraintForceX=off  SenseConstraintForceY=off  SenseConstraintForceZ=off  SenseConstraintTorque=off  SenseConstraintTorqueX=off  SenseConstraintTorqueY=off  SenseConstraintTorqueZ=off  SenseTotalForce=off  SenseTotalForceX=off  SenseTotalForceY=off  SenseTotalForceZ=off  SenseTotalTorque=off  SenseTotalTorqueX=off  SenseTotalTorqueY=off  SenseTotalTorqueZ=off  CompositeWrenchDir=FollowerOnBase  CompositeWrenchFrame=BaseFrame  EquilibriumPosition=0  EquilibriumPositionUnits=deg  SpringStiffness=stif_rot  SpringStiffnessUnits=N*m/rad  DampingCoefficient=0  DampingCoefficientUnits=N*m/(rad/s)  TorqueActuationMode=InputTorque  MotionActuationMode=ComputedMotion  SensePosition=on  SenseVelocity=on  SenseAcceleration=off  SenseTorqueForce=off  SenseLowerLimitTorqueForce=off  SenseUpperLimitTorqueForce=off  LowerLimitSpecify=on  LowerLimitBound=-45  LowerLimitBoundUnits=deg  LowerLimitStiffness=stif_m  LowerLimitStiffnessUnits=N*m/rad  LowerLimitDamping=damp_m  LowerLimitDampingUnits=N*m/(rad/s)  LowerLimitTransitionRegionWidth=0.1  LowerLimitTransitionRegionWidthUnits=deg  UpperLimitSpecify=on  UpperLimitBound=45  UpperLimitBoundUnits=deg  UpperLimitStiffness=stif_m  UpperLimitStiffnessUnits=N*m/rad  UpperLimitDamping=damp_m  UpperLimitDampingUnits=N*m/(rad/s)  UpperLimitTransitionRegionWidth=0.1  UpperLimitTransitionRegionWidthUnits=deg  PositionTargetSpecify=off  PositionTargetPriority=High  PositionTargetValue=20  PositionTargetValueUnits=deg  VelocityTargetSpecify=off  VelocityTargetPriority=High  VelocityTargetValue=0  VelocityTargetValueUnits=deg/s
  Scope1 : Scope
  Stroke Joint : sm_lib/Joints/Revolute Joint  JointMode=Normal  SenseConstraintForce=off  SenseConstraintForceX=off  SenseConstraintForceY=off  SenseConstraintForceZ=off  SenseConstraintTorque=off  SenseConstraintTorqueX=off  SenseConstraintTorqueY=off  SenseConstraintTorqueZ=off  SenseTotalForce=off  SenseTotalForceX=off  SenseTotalForceY=off  SenseTotalForceZ=off  SenseTotalTorque=off  SenseTotalTorqueX=off  SenseTotalTorqueY=off  SenseTotalTorqueZ=off  CompositeWrenchDir=FollowerOnBase  CompositeWrenchFrame=BaseFrame  EquilibriumPosition=0  EquilibriumPositionUnits=deg  SpringStiffness=0  SpringStiffnessUnits=N*m/deg  DampingCoefficient=0  DampingCoefficientUnits=N*m/(deg/s)  TorqueActuationMode=ComputedTorque  MotionActuationMode=InputMotion  SensePosition=on  SenseVelocity=on  SenseAcceleration=off  SenseTorqueForce=off  SenseLowerLimitTorqueForce=off  SenseUpperLimitTorqueForce=off  LowerLimitSpecify=on  LowerLimitBound=-90  LowerLimitBoundUnits=deg  LowerLimitStiffness=1e4  LowerLimitStiffnessUnits=N*m/deg  LowerLimitDamping=10  LowerLimitDampingUnits=N*m/(deg/s)  LowerLimitTransitionRegionWidth=0.1  LowerLimitTransitionRegionWidthUnits=deg  UpperLimitSpecify=on  UpperLimitBound=90  UpperLimitBoundUnits=deg  UpperLimitStiffness=1e4  UpperLimitStiffnessUnits=N*m/deg  UpperLimitDamping=10  UpperLimitDampingUnits=N*m/(deg/s)  UpperLimitTransitionRegionWidth=0.1  UpperLimitTransitionRegionWidthUnits=deg  PositionTargetSpecify=off  PositionTargetPriority=High  PositionTargetValue=-30  PositionTargetValueUnits=deg  VelocityTargetSpecify=off  VelocityTargetPriority=High  VelocityTargetValue=0  VelocityTargetValueUnits=deg/s
  To Workspace : ToWorkspace  VariableName=t  SampleTime=-1
  move r_cp : sm_lib/Frames and Transforms/Rigid Transform  TranslationMethod=Cartesian  TranslationStandardOffset=r_cp  TranslationLengthUnit=m  TranslationStandardAxis=+Y  TranslationCartesianOffset=[0 r_cp 0]  TranslationROffset=0  TranslationROffsetUnits=m  TranslationZOffset=0  TranslationZOffsetUnits=m  TranslationThetaOffset=0  TranslationThetaOffsetUnits=deg  RotationMethod=None  RotationAngleUnits=deg  RotationStandardAxis=+Y  RotationAngle=90  RotationArbitraryAxis=[0 0 1]  FollAlignAxisA=+X  BaseAlignAxisA=+Y  FollAlignAxisB=+Y  BaseAlignAxisB=+Z  RotationSequenceAxes=FollowerAxes  RotationSequence=XYX  RotationSequenceAngles=[0 0 0]  RotationSequenceAnglesUnits=deg  RotationMatrix=[1 0 0; 0 1 0; 0 0 1]
  z-y1 : sm_lib/Frames and Transforms/Rigid Transform  TranslationMethod=None  TranslationStandardOffset=0  TranslationLengthUnit=cm  TranslationStandardAxis=+Z  TranslationCartesianOffset=[0 1 4]  TranslationROffset=0  TranslationROffsetUnits=m  TranslationZOffset=0  TranslationZOffsetUnits=m  TranslationThetaOffset=0  TranslationThetaOffsetUnits=deg  RotationMethod=StandardAxis  RotationAngleUnits=deg  RotationStandardAxis=+X  RotationAngle=90  RotationArbitraryAxis=[0 0 1]  FollAlignAxisA=+X  BaseAlignAxisA=+Y  FollAlignAxisB=+Y  BaseAlignAxisB=+Z  RotationSequenceAxes=FollowerAxes  RotationSequence=XYX  RotationSequenceAngles=[0 0 0]  RotationSequenceAnglesUnits=deg  RotationMatrix=[0 0 1; 1 0 0; 0 1 0]
  q of Left Stroke : PMIOPort  Side=Left
  FN of Left : PMIOPort  Port=2  Side=Left
  T of Left : PMIOPort  Port=3  Side=Left
  LT : PMIOPort  Port=4  Side=Left
  d_cp : PMIOPort  Port=5  Side=Left
  Meas : PMIOPort  Port=6  Side=Right
  Out Bus Element5 : Outport  PortName=left  Element=stroke
  Out Bus Element6 : Outport  PortName=left  Element=stroke_vel
  Out Bus Element7 : Outport  PortName=left  Element=rotate
  Out Bus Element1 : Outport  PortName=left  Element=rotate_vel
  wires:
  PS-Simulink Converter13/1 -> [psi_l]
  PS-Simulink Converter17/1 -> [psi_dot_l]
  PS-Simulink Converter14/1 -> [theta_l]
  [psi_dot_l] -> Out Bus Element6/1
  [psi_l] -> Out Bus Element5/1
  [theta_l] -> Out Bus Element7/1
  PS-Simulink Converter1/1 -> [theta_dot_l]
  [theta_dot_l] -> Out Bus Element1/1
  Clock/1 -> Scope1/1, To Workspace/1
  connections:
  Stroke Joint/RConn2 -- PS-Simulink Converter13/LConn1
  Stroke Joint/RConn3 -- PS-Simulink Converter17/LConn1
  Revolute Joint/RConn1 -- z-y1/LConn1
  Stroke Joint/LConn1 -- LT/RConn1
  Stroke Joint/RConn1 -- Left LE/LConn1
  Revolute Joint/RConn2 -- PS-Simulink Converter14/LConn1
  Stroke Joint/LConn2 -- q of Left Stroke/RConn1
  Revolute Joint/LConn1 -- Left LE/RConn1
  Revolute Joint/RConn3 -- PS-Simulink Converter1/LConn1
  T of Left/RConn1 -- Revolute Joint/LConn2
  Graphic/RConn1 -- Prismatic Joint/RConn1 -- External Force and Torque/RConn1
  FN of Left/RConn1 -- External Force and Torque/LConn1
  d_cp/RConn1 -- Prismatic Joint/LConn2
  Prismatic Joint/LConn1 -- move r_cp/RConn1
  Left Wing1/LConn1 -- Meas/RConn1 -- z-y1/RConn1 -- move r_cp/LConn1

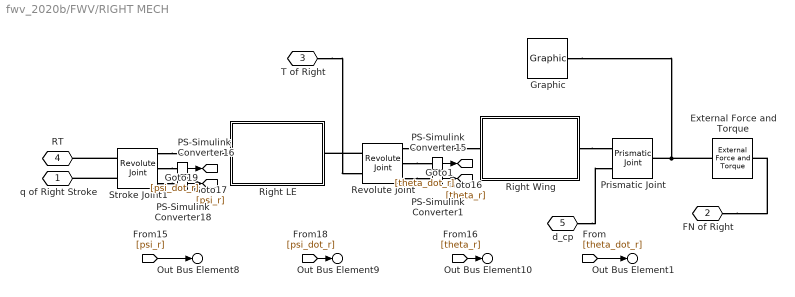
== system fwv_2020b/FWV/RIGHT MECH ==
  External Force and Torque : sm_lib/Forces and Torques/External Force and Torque  ForceResolutionFrame=AttachedFrame  EnableForceX=on  EnableForceY=off  EnableForceZ=off  EnableForce=off  TorqueResolutionFrame=AttachedFrame  EnableTorqueX=off  EnableTorqueY=off  EnableTorqueZ=off  EnableTorque=off
  Graphic : sm_lib/Body Elements/Graphic  GraphicType=Marker  MarkerShape=Frame  MarkerSize=20  GraphicVisPropType=SimpleVisualProperties  GraphicDiffuseColor=[1 0 1]  GraphicSpecularColor=[0.5 0.5 0.5 1.0]  GraphicAmbientColor=[0.15 0.15 0.15 1.0]  GraphicEmissiveColor=[0.0 0.0 0.0 1.0]  GraphicShininess=75  GraphicOpacity=1.0
  PS-Simulink Converter{1,15..16,18} (4 alike) : nesl_utility/PS-Simulink Converter  PhysicalDomain=network_engine_domain  SubClassName=ps_output  LeftPortType=input  RightPortType=output  PseudoPeriodic=off  Frequencies=[]  Unit=inherit  AffineConversion=off
      settings: SourceProductBaseCode=PW,SS
  Prismatic Joint : sm_lib/Joints/Prismatic Joint  JointMode=Normal  SenseConstraintForce=off  SenseConstraintForceX=off  SenseConstraintForceY=off  SenseConstraintForceZ=off  SenseConstraintTorque=off  SenseConstraintTorqueX=off  SenseConstraintTorqueY=off  SenseConstraintTorqueZ=off  SenseTotalForce=off  SenseTotalForceX=off  SenseTotalForceY=off  SenseTotalForceZ=off  SenseTotalTorque=off  SenseTotalTorqueX=off  SenseTotalTorqueY=off  SenseTotalTorqueZ=off  CompositeWrenchDir=FollowerOnBase  CompositeWrenchFrame=BaseFrame  EquilibriumPosition=0  EquilibriumPositionUnits=m  SpringStiffness=0  SpringStiffnessUnits=N/m  DampingCoefficient=0  DampingCoefficientUnits=N/(m/s)  TorqueActuationMode=ComputedTorque  MotionActuationMode=InputMotion  SensePosition=off  SenseVelocity=off  SenseAcceleration=off  SenseTorqueForce=off  SenseLowerLimitTorqueForce=off  SenseUpperLimitTorqueForce=off  LowerLimitSpecify=off  LowerLimitBound=-1  LowerLimitBoundUnits=m  LowerLimitStiffness=1e6  LowerLimitStiffnessUnits=N/m  LowerLimitDamping=1e3  LowerLimitDampingUnits=N/(m/s)  LowerLimitTransitionRegionWidth=1e-4  LowerLimitTransitionRegionWidthUnits=m  UpperLimitSpecify=off  UpperLimitBound=1  UpperLimitBoundUnits=m  UpperLimitStiffness=1e6  UpperLimitStiffnessUnits=N/m  UpperLimitDamping=1e3  UpperLimitDampingUnits=N/(m/s)  UpperLimitTransitionRegionWidth=1e-4  UpperLimitTransitionRegionWidthUnits=m  PositionTargetSpecify=off  PositionTargetPriority=High  PositionTargetValue=0  PositionTargetValueUnits=m  VelocityTargetSpecify=off  VelocityTargetPriority=High  VelocityTargetValue=0  VelocityTargetValueUnits=m/s
  Revolute Joint : sm_lib/Joints/Revolute Joint  JointMode=Normal  SenseConstraintForce=off  SenseConstraintForceX=off  SenseConstraintForceY=off  SenseConstraintForceZ=off  SenseConstraintTorque=off  SenseConstraintTorqueX=off  SenseConstraintTorqueY=off  SenseConstraintTorqueZ=off  SenseTotalForce=off  SenseTotalForceX=off  SenseTotalForceY=off  SenseTotalForceZ=off  SenseTotalTorque=off  SenseTotalTorqueX=off  SenseTotalTorqueY=off  SenseTotalTorqueZ=off  CompositeWrenchDir=FollowerOnBase  CompositeWrenchFrame=BaseFrame  EquilibriumPosition=0  EquilibriumPositionUnits=deg  SpringStiffness=stif_rot  SpringStiffnessUnits=N*m/rad  DampingCoefficient=0  DampingCoefficientUnits=N*m/(rad/s)  TorqueActuationMode=InputTorque  MotionActuationMode=ComputedMotion  SensePosition=on  SenseVelocity=on  SenseAcceleration=off  SenseTorqueForce=off  SenseLowerLimitTorqueForce=off  SenseUpperLimitTorqueForce=off  LowerLimitSpecify=on  LowerLimitBound=-45  LowerLimitBoundUnits=deg  LowerLimitStiffness=stif_m  LowerLimitStiffnessUnits=N*m/rad  LowerLimitDamping=damp_m  LowerLimitDampingUnits=N*m/(rad/s)  LowerLimitTransitionRegionWidth=0.1  LowerLimitTransitionRegionWidthUnits=deg  UpperLimitSpecify=on  UpperLimitBound=45  UpperLimitBoundUnits=deg  UpperLimitStiffness=stif_m  UpperLimitStiffnessUnits=N*m/rad  UpperLimitDamping=damp_m  UpperLimitDampingUnits=N*m/(rad/s)  UpperLimitTransitionRegionWidth=0.1  UpperLimitTransitionRegionWidthUnits=deg  PositionTargetSpecify=off  PositionTargetPriority=High  PositionTargetValue=20  PositionTargetValueUnits=deg  VelocityTargetSpecify=off  VelocityTargetPriority=High  VelocityTargetValue=0  VelocityTargetValueUnits=deg/s
  Right LE : Subsystem
  Right Wing : Subsystem
  Stroke Joint1 : sm_lib/Joints/Revolute Joint  JointMode=Normal  SenseConstraintForce=off  SenseConstraintForceX=off  SenseConstraintForceY=off  SenseConstraintForceZ=off  SenseConstraintTorque=off  SenseConstraintTorqueX=off  SenseConstraintTorqueY=off  SenseConstraintTorqueZ=off  SenseTotalForce=off  SenseTotalForceX=off  SenseTotalForceY=off  SenseTotalForceZ=off  SenseTotalTorque=off  SenseTotalTorqueX=off  SenseTotalTorqueY=off  SenseTotalTorqueZ=off  CompositeWrenchDir=FollowerOnBase  CompositeWrenchFrame=BaseFrame  EquilibriumPosition=0  EquilibriumPositionUnits=deg  SpringStiffness=0  SpringStiffnessUnits=N*m/deg  DampingCoefficient=0  DampingCoefficientUnits=N*m/(deg/s)  TorqueActuationMode=ComputedTorque  MotionActuationMode=InputMotion  SensePosition=on  SenseVelocity=on  SenseAcceleration=off  SenseTorqueForce=off  SenseLowerLimitTorqueForce=off  SenseUpperLimitTorqueForce=off  LowerLimitSpecify=on  LowerLimitBound=-90  LowerLimitBoundUnits=deg  LowerLimitStiffness=1e4  LowerLimitStiffnessUnits=N*m/deg  LowerLimitDamping=10  LowerLimitDampingUnits=N*m/(deg/s)  LowerLimitTransitionRegionWidth=0.1  LowerLimitTransitionRegionWidthUnits=deg  UpperLimitSpecify=on  UpperLimitBound=90  UpperLimitBoundUnits=deg  UpperLimitStiffness=1e4  UpperLimitStiffnessUnits=N*m/deg  UpperLimitDamping=10  UpperLimitDampingUnits=N*m/(deg/s)  UpperLimitTransitionRegionWidth=0.1  UpperLimitTransitionRegionWidthUnits=deg  PositionTargetSpecify=on  PositionTargetPriority=High  PositionTargetValue=30  PositionTargetValueUnits=deg  VelocityTargetSpecify=off  VelocityTargetPriority=High  VelocityTargetValue=0  VelocityTargetValueUnits=deg/s
  q of Right Stroke : PMIOPort  Side=Left
  FN of Right : PMIOPort  Port=2  Side=Left
  T of Right : PMIOPort  Port=3  Side=Left
  RT : PMIOPort  Port=4  Side=Left
  d_cp : PMIOPort  Port=5  Side=Left
  Out Bus Element8 : Outport  PortName=right  Element=stroke
  Out Bus Element9 : Outport  PortName=right  Element=stroke_vel
  Out Bus Element10 : Outport  PortName=right  Element=rotate
  Out Bus Element1 : Outport  PortName=right  Element=rotate_vel
  wires:
  PS-Simulink Converter15/1 -> [theta_r]
  PS-Simulink Converter18/1 -> [psi_dot_r]
  PS-Simulink Converter16/1 -> [psi_r]
  [psi_r] -> Out Bus Element8/1
  [theta_r] -> Out Bus Element10/1
  [psi_dot_r] -> Out Bus Element9/1
  PS-Simulink Converter1/1 -> [theta_dot_r]
  [theta_dot_r] -> Out Bus Element1/1
  connections:
  Revolute Joint/RConn2 -- PS-Simulink Converter15/LConn1
  Stroke Joint1/LConn1 -- RT/RConn1
  Stroke Joint1/RConn3 -- PS-Simulink Converter18/LConn1
  Stroke Joint1/LConn2 -- q of Right Stroke/RConn1
  Revolute Joint/LConn1 -- Right LE/RConn1
  Revolute Joint/RConn1 -- Right Wing/LConn1
  Stroke Joint1/RConn1 -- Right LE/LConn1
  Stroke Joint1/RConn2 -- PS-Simulink Converter16/LConn1
  Revolute Joint/RConn3 -- PS-Simulink Converter1/LConn1
  Graphic/RConn1 -- External Force and Torque/RConn1 -- Prismatic Joint/RConn1
  Right Wing/RConn1 -- Prismatic Joint/LConn1
  FN of Right/RConn1 -- External Force and Torque/LConn1
  d_cp/RConn1 -- Prismatic Joint/LConn2
  T of Right/RConn1 -- Revolute Joint/LConn2
